simulink model "Simple"
settings: Solver=ode45  SolverMode=SingleTasking  StartTime=0.0  StopTime=10.0  RelTol=1e-3
settings Model: Creator=Student  LastModifiedBy=Student
settings DataIOCC: LimitDataPoints=on  SaveFormat=Array  SignalLoggingSaveFormat=ModelDataLogs  ReturnWorkspaceOutputs=off
settings OptimizationCC: BlockReduction=off  BooleanDataType=off  ExpressionDepthLimit=2147483647  LifeSpan=inf  SimCompilerOptimization=Off
settings DebuggingCC: SaveWithParameterizedLinksMsg=none  UnderspecifiedInitializationDetection=Classic  MergeDetectMultiDrivingBlocksExec=none  SignalResolutionControl=TryResolveAllWithWarning  MultiTaskDSMMsg=warning  MultiTaskCondExecSysMsg=none  FcnCallInpInsideContextMsg=Enable All  FrameProcessingCompatibilityMsg=warning  StateNameClashWarn=warning  StrictBusMsg=None  SFUnexpectedBacktrackingDiag=warning  SFNoUnconditionalDefaultTransitionDiag=warning
settings HardwareCC: ProdBitPerPointer=32  ProdLargestAtomicFloat=None  ProdIntDivRoundTo=Undefined  ProdEndianess=Unspecified  ProdWordSize=32  ProdHWDeviceType=32-bit Generic  TargetUnknown=on
settings ModelReferenceCC: PropagateSignalLabelsOutOfModel=off
settings SFSimCC: SimUseLocalCustomCode=off
settings RTWCC: RTWUseLocalCustomCode=off  IncludeERTFirstTime=on  RTWCompilerOptimization=Off
settings CodeAppCC: CustomSymbolStrType=$N$R$M
settings GRTTargetCC: CodeReplacementLibrary=ANSI_C  GeneratePreprocessorConditionals=Disable all  CPPClassGenCompliant=off

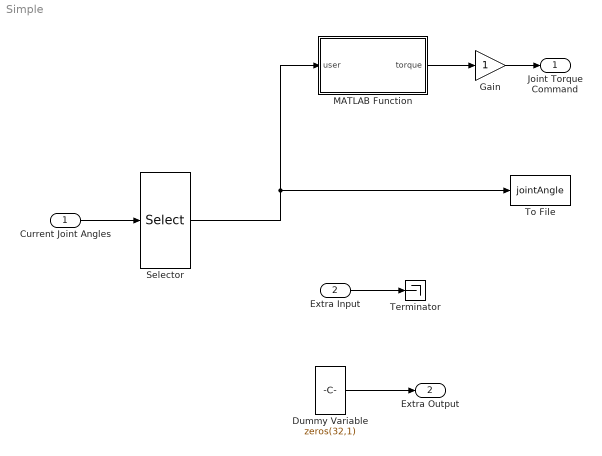
== system Simple ==
  Current Joint Angles : Inport  PortDimensions=6
  Extra Input : Inport  Port=2  PortDimensions=16
  Dummy Variable : Constant  Value=zeros(32,1)
  Gain : Gain
  MATLAB Function : MATLAB Function  TreatAsAtomicUnit=on
  Selector : Selector  InputPortWidth=6  IndexOptions=Index vector (dialog)  Indices=1:3  OutputSizes=1
  Terminator : Terminator
  To File : ToFile  Filename=jointAngle  MatrixName=tq
  Joint Torque Command : Outport  PortDimensions=3
  Extra Output : Outport  Port=2  PortDimensions=32
  wires:
  Current Joint Angles/1 -> Selector/1
  Selector/1 -> To File/1, MATLAB Function/1(user)
  Dummy Variable/1 -> Extra Output/1
  Extra Input/1 -> Terminator/1
  Gain/1 -> Joint Torque Command/1
  MATLAB Function/1(torque) -> Gain/1

== matlab function Simple/MATLAB Function ==
  data: user input; torque output
function torque = haptic_control(user)
c = [0;0;0];
r = 30;

des_pos = c;
curr_pos = OmniForwardKinematics(user);
error = des_pos - curr_pos;
J = Omnijacobian(user);

if error >= r
    torque = J'*error;
else
    torque = c;
end
end
